simulink model "segway_simulink"  (R2021b)
settings: Solver=VariableStepAuto  StartTime=0.0  StopTime=5  FixedStep=a  RelTol=1e-3
values from neighbouring files (symbols this model uses):
  A = [0         1         0          0 ... (first row only)    [Segway_Init.m]
  b = [ 0 ... (first row only)    [Segway_Init.m]
  F = 1/(cts*(-A+b*K)^-1*b)    [Segway_Init.m]
  K = lqr(A,b,Q,R)    [Segway_Init.m]
settings Model: Creator=Hot  LastModifiedBy=Hot

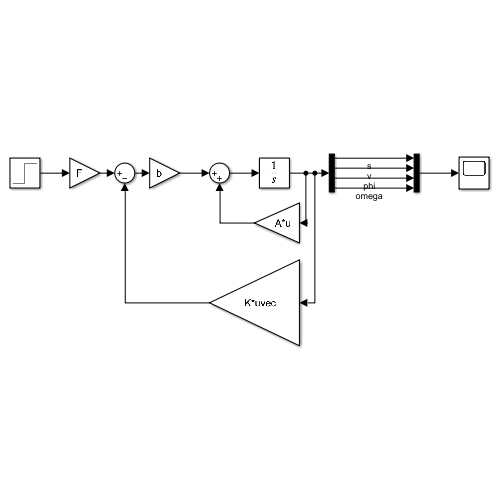
[thumbnail: Simulink's stored preview of the top-level diagram]
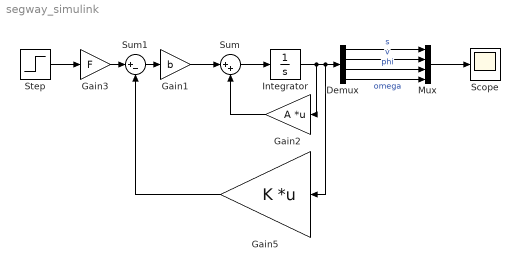
== system segway_simulink ==
  Demux : Demux
  Gain1 : Gain  Gain=b
  Gain2 : Gain  Gain=A  Multiplication=Matrix(K*u)
  Gain3 : Gain  Gain=F
  Gain5 : Gain  Gain=K  Multiplication=Matrix(K*u) (u vector)
  Integrator : Integrator
  Mux : Mux
  Scope : Scope
  Step : Step  Time=0.1  SampleTime=0
  Sum : Sum  Inputs=|++
  Sum1 : Sum  Inputs=|+-
  wires:
  Integrator/1 -> Gain2/1, Gain5/1, Demux/1
  Demux/2 -> Mux/2  "v"
  Demux/1 -> Mux/1  "s"
  Demux/3 -> Mux/3  "phi"
  Demux/4 -> Mux/4  "omega"
  Mux/1 -> Scope/1
  Sum/1 -> Integrator/1
  Gain1/1 -> Sum/1
  Gain2/1 -> Sum/2
  Step/1 -> Gain3/1
  Gain3/1 -> Sum1/1
  Sum1/1 -> Gain1/1
  Gain5/1 -> Sum1/2
